simulink model "mil_top_atc"  (R2025b)
settings: Solver=FixedStepDiscrete  StartTime=0.0  StopTime=mil_atc_t_final_s  FixedStep=0.01  RelTol=1e-3
settings Model: Creator=O.Agaphonov  LastModifiedBy=O.Agaphonov

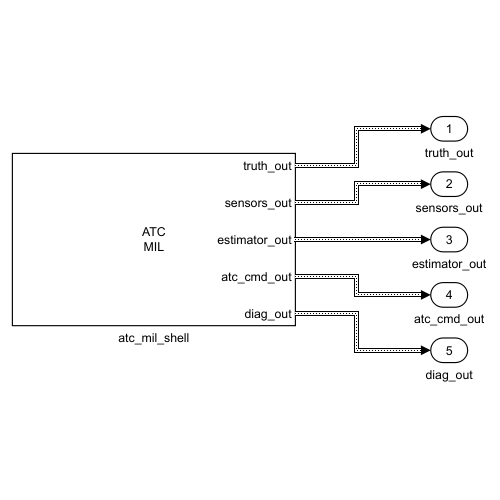
[thumbnail: Simulink's stored preview of the top-level diagram]
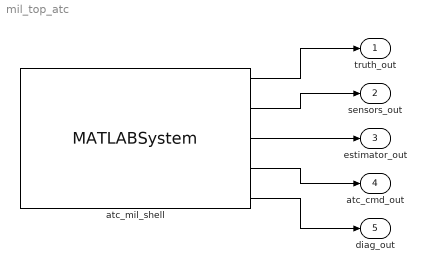
== system mil_top_atc ==
  atc_mil_shell : MATLABSystem  System=uav.sl.Stage15ATCMILSystem  dt_s=mil_atc_dt_s  params=mil_atc_params  state0=mil_atc_state0  bridge_cfg=mil_atc_bridge_cfg  time_s=0.0  SimulateUsing=Interpreted execution
      mask Type: uav.sl.Stage15ATCMILSystem
  truth_out : Outport
  sensors_out : Outport  Port=2
  estimator_out : Outport  Port=3
  atc_cmd_out : Outport  Port=4
  diag_out : Outport  Port=5
  wires:
  atc_mil_shell/1 -> truth_out/1
  atc_mil_shell/2 -> sensors_out/1
  atc_mil_shell/3 -> estimator_out/1
  atc_mil_shell/4 -> atc_cmd_out/1
  atc_mil_shell/5 -> diag_out/1
